simulink model "test_dynamics"  (R2016a)
settings: Solver=VariableStepAuto  StartTime=0.0  StopTime=10.0  RelTol=1e-3
settings Model: Creator=andreanv  LastModifiedBy=andreanv

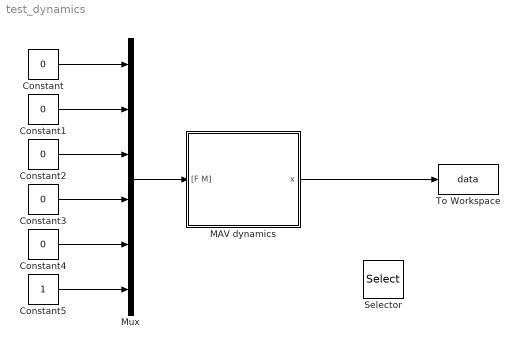
== system test_dynamics ==
  Constant{,1..4} (5 alike) : Constant  Value=0
  Constant5 : Constant
  MAV dynamics : Subsystem
  Mux : Mux  Inputs=6
  Selector : Selector  InputPortWidth=12  IndexOptions=Index vector (dialog)  Indices=[1:9]  OutputSizes=1
  To Workspace : ToWorkspace  VariableName=data  SaveFormat=Timeseries  SampleTime=-1
  wires:
  Constant5/1 -> Mux/6
  Constant4/1 -> Mux/5
  Constant3/1 -> Mux/4
  Constant1/1 -> Mux/2
  Constant2/1 -> Mux/3
  Constant/1 -> Mux/1
  Mux/1 -> MAV dynamics/1("[F M]")
  MAV dynamics/1(x) -> To Workspace/1

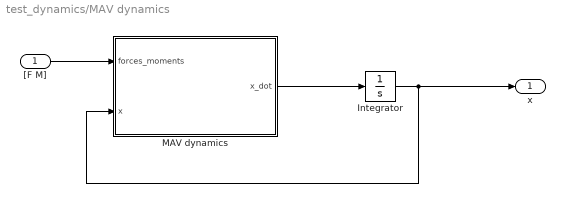
== system test_dynamics/MAV dynamics ==
  "[F M]" : Inport  OutMin=[6]  OutMax=[6]
  Integrator : Integrator  InitialCondition=[0;0;0;0;0;0;0;0;0;0;0;0]
  MAV dynamics : MATLAB Function  TreatAsAtomicUnit=on
  x : Outport
  wires:
  Integrator/1 -> x/1, MAV dynamics/2(x)
  "[F M]"/1 -> MAV dynamics/1(forces_moments)
  MAV dynamics/1(x_dot) -> Integrator/1

== matlab function test_dynamics/MAV dynamics/MAV dynamics ==
  data: forces_moments input; x_dot output; x input; P parameter
function x_dot = fcn(forces_moments, x, P)

    x_dot = mav_dynamics(forces_moments, x, P);
    
end
